simulink subsystem "Ss_controller__robust_integral"  (R2024b)
settings: Solver=VariableStepAuto  StartTime=0.0  StopTime=10.0  RelTol=1e-3
values from neighbouring files (symbols this model uses):
  K_stateFB = place(Ae, Be, poles)    [Controller_StateSpace_Lab1.m]
  Nu = Sol(3, :)    [Controller_StateSpace_Lab1.m]
  Nx = Sol(1:2, :)    [Controller_StateSpace_Lab1.m]
  rpm2rads = 2*pi/60    (= 0.10471975512)    [Plant_EstimTrialUpdateLAB17_04_25.m]
settings Model: Creator=Utente  LastModifiedBy=Buton

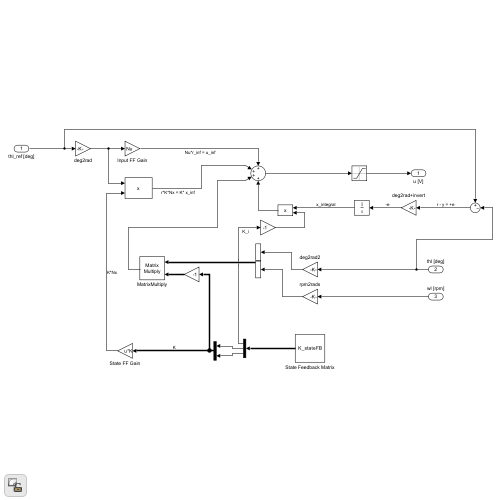
[thumbnail: Simulink's stored preview of the top-level diagram]
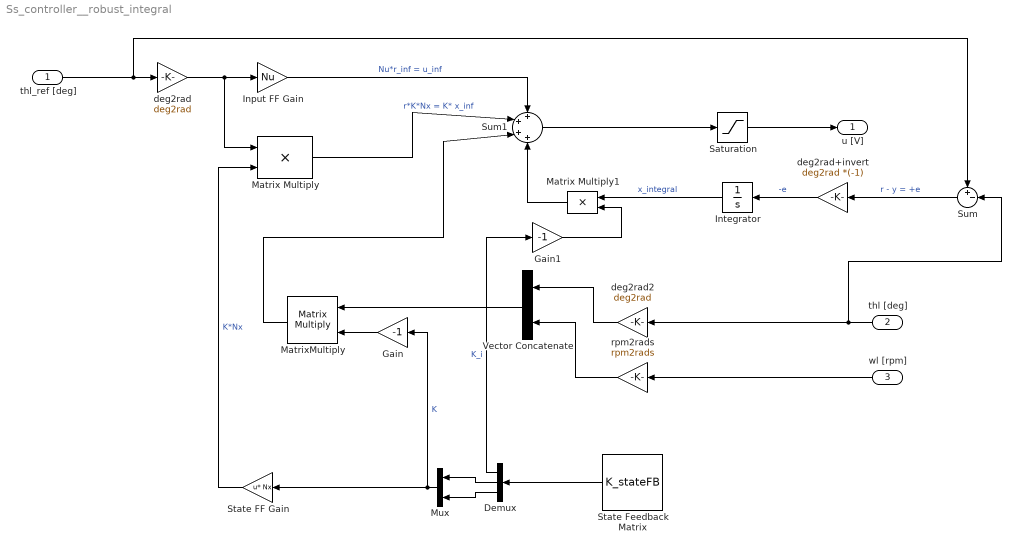
== system Ss_controller__robust_integral ==
  thl_ref [deg] : Inport
  thl [deg] : Inport  Port=2
  wl [rpm] : Inport  Port=3
  Demux : Demux  Outputs=3
  Gain : Gain  Gain=-1
  Gain1 : Gain  Gain=-1
  Input FF Gain : Gain  Gain=Nu
  Integrator : Integrator
  Matrix Multiply : Product
  Matrix Multiply1 : Product
  MatrixMultiply : Product  Multiplication=Matrix(*)
  Mux : Mux  Inputs=2
  Saturation : Saturate  UpperLimit=12  LowerLimit=-12
  State FF Gain : Gain  Gain=Nx  Multiplication=Matrix(u*K)
  State Feedback Matrix : Constant  Value=K_stateFB
  Sum : Sum  Inputs=+-|
  Sum1 : Sum  Inputs=++++
  Vector Concatenate : Concatenate
  deg2rad : Gain  Gain=deg2rad
  deg2rad+invert : Gain  Gain=deg2rad *(-1)
  deg2rad2 : Gain  Gain=deg2rad
  rpm2rads : Gain  Gain=rpm2rads
  u [V] : Outport
  wires:
  Sum1/1 -> Saturation/1
  thl_ref [deg]/1 -> deg2rad/1, Sum/1
  deg2rad2/1 -> Vector Concatenate/1
  Saturation/1 -> u [V]/1
  deg2rad/1 -> Input FF Gain/1, Matrix Multiply/1
  Input FF Gain/1 -> Sum1/1  "Nu*r_inf = u_inf"
  rpm2rads/1 -> Vector Concatenate/2
  State FF Gain/1 -> Matrix Multiply/2  "K*Nx"
  Matrix Multiply/1 -> Sum1/2  "r*K*Nx = K* x_inf"
  Gain/1 -> MatrixMultiply/2
  Vector Concatenate/1 -> MatrixMultiply/1
  MatrixMultiply/1 -> Sum1/3
  Sum/1 -> deg2rad+invert/1  "r - y = +e"
  wl [rpm]/1 -> rpm2rads/1
  thl [deg]/1 -> Sum/2, deg2rad2/1
  State Feedback Matrix/1 -> Demux/1
  Matrix Multiply1/1 -> Sum1/4
  Integrator/1 -> Matrix Multiply1/1  "x_integral"
  Demux/1 -> Gain1/1  "K_i"
  Demux/2 -> Mux/1
  Demux/3 -> Mux/2
  Mux/1 -> State FF Gain/1, Gain/1  "K"
  Gain1/1 -> Matrix Multiply1/2
  deg2rad+invert/1 -> Integrator/1  "-e"
